simulink model "commande_position_axe"  (R2024b)
settings: Solver=VariableStepAuto  StartTime=0.0  StopTime=10.0  RelTol=1e-3
settings Model: Creator=firas  LastModifiedBy=firas

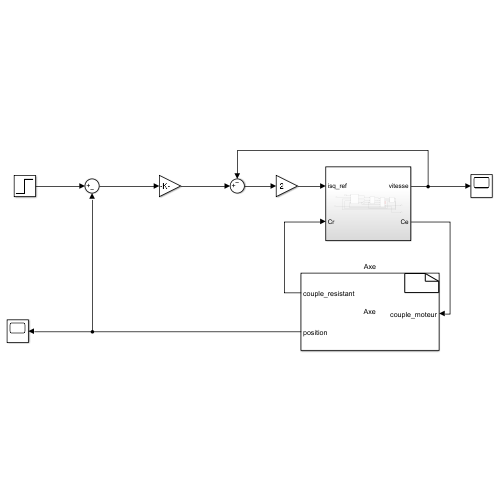
[thumbnail: Simulink's stored preview of the top-level diagram]
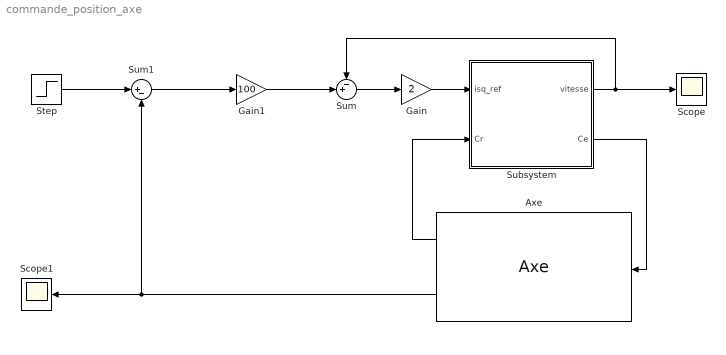
== system commande_position_axe ==
  Axe : S-Function  FunctionName=Axe  SFunctionModules=Axe_wrapper.c  SFunctionDeploymentMode=off  EnableBusSupport=off  mask(S-Function Builder){}
      mask help: Simulink:masks:SFunctionBuilder_MD
      mask init:
      | val = [[.9  0.75 0.75 1 1 .9 .9 1]',[1 1 0.75 0.75 .9 .9 1 .9]'];try , sys = get_param(gcb,'SfunBuilderFcnName');if isempty(sys), sys = get_param(gcb,'FunctionName'); end,catch, sys = get_param(gcb,'FunctionName'); end
      settings: CopyFcn=set_param(gcbh,'LinkStatus','none')  OpenFcn=sfunctionwizard(gcbh)
      mask Display:
      | plot(val(:,1),val(:,2))
      | disp(sys)
      | port_label('input',1,sprintf('%s', 'couple\_moteur'),'interpreter','tex')
      | port_label('output',1,sprintf('%s', 'couple\_resistant'),'interpreter','tex')
      | port_label('output',2,sprintf('%s', 'position'),'interpreter','tex')
  Gain : Gain  Gain=2
  Gain1 : Gain  Gain=100
  Scope : Scope
  Scope1 : Scope
  Step : Step  SampleTime=0
  Subsystem : Subsystem
  Sum : Sum  Inputs=-+|
  Sum1 : Sum  Inputs=|+-
  wires:
  Subsystem/2(Ce) -> Axe/1
  Axe/1 -> Subsystem/2(Cr)
  Sum/1 -> Gain/1
  Gain/1 -> Subsystem/1(isq_ref)
  Subsystem/1(vitesse) -> Scope/1, Sum/1
  Step/1 -> Sum1/1
  Axe/2 -> Sum1/2, Scope1/1
  Sum1/1 -> Gain1/1
  Gain1/1 -> Sum/2

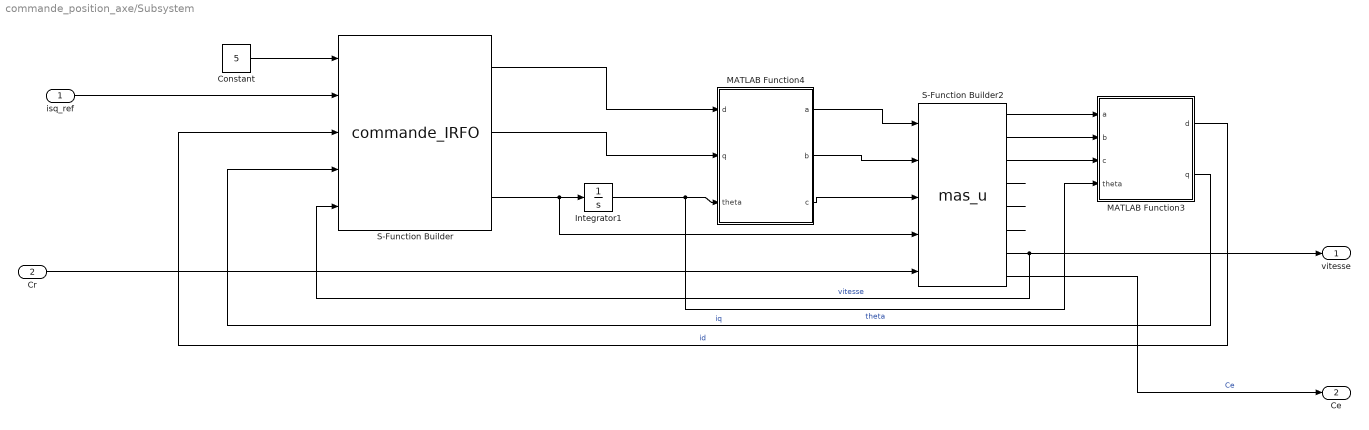
== system commande_position_axe/Subsystem ==
  isq_ref : Inport
  Cr : Inport  Port=2
  Constant : Constant  Value=5
  Integrator1 : Integrator
  MATLAB Function3 : MATLAB Function  TreatAsAtomicUnit=on
  MATLAB Function4 : MATLAB Function  TreatAsAtomicUnit=on
  S-Function Builder : S-Function  FunctionName=commande_IRFO  SFunctionModules=commande_IRFO_wrapper.c  SFunctionDeploymentMode=off  EnableBusSupport=off  mask(S-Function Builder){}
      mask help: Simulink:masks:SFunctionBuilder_MD
      mask init: same as commande_position_axe/Axe
      settings: CopyFcn=set_param(gcbh,'LinkStatus','none')  OpenFcn=sfunctionwizard(gcbh)
      mask Display:
      | plot(val(:,1),val(:,2))
      | disp(sys)
      | port_label('input',1,sprintf('%s', 'iphi\_ref'),'interpreter','tex')
      | port_label('input',2,sprintf('%s', 'isq\_ref'),'interpreter','tex')
      | port_label('input',3,sprintf('%s', 'isd'),'interpreter','tex')
      | port_label('input',4,sprintf('%s', 'isq'),'interpreter','tex')
      | port_label('input',5,sprintf('%s', 'vitesse'),'interpreter','tex')
      | port_label('output',1,sprintf('%s', 'vsd'),'interpreter','tex')
      | port_label('output',2,sprintf('%s', 'vsq'),'interpreter','tex')
      | port_label('output',3,sprintf('%s', 'ws'),'interpreter','tex')
  S-Function Builder2 : S-Function  FunctionName=mas_u  SFunctionModules=mas_u_wrapper.c  SFunctionDeploymentMode=off  EnableBusSupport=off  mask(S-Function Builder){}
      mask help: Simulink:masks:SFunctionBuilder_MD
      mask init: same as commande_position_axe/Axe
      settings: CopyFcn=set_param(gcbh,'LinkStatus','none')  OpenFcn=sfunctionwizard(gcbh)
      mask Display:
      | plot(val(:,1),val(:,2))
      | disp(sys)
      | port_label('input',1,sprintf('%s', 'vsa'),'interpreter','tex')
      | port_label('input',2,sprintf('%s', 'vsb'),'interpreter','tex')
      | port_label('input',3,sprintf('%s', 'vsc'),'interpreter','tex')
      | port_label('input',4,sprintf('%s', 'ws'),'interpreter','tex')
      | port_label('input',5,sprintf('%s', 'Cr'),'interpreter','tex')
      | port_label('output',1,sprintf('%s', 'isa'),'interpreter','tex')
      | port_label('output',2,sprintf('%s', 'isb'),'interpreter','tex')
      | port_label('output',3,sprintf('%s', 'isc'),'interpreter','tex')
      | port_label('output',4,sprintf('%s', 'ira'),'interpreter','tex')
      | port_label('output',5,sprintf('%s', 'irb'),'interpreter','tex')
      | port_label('output',6,sprintf('%s', 'irc'),'interpreter','tex')
      | port_label('output',7,sprintf('%s', 'vitesse'),'interpreter','tex')
      | port_label('output',8,sprintf('%s', 'Ce'),'interpreter','tex')
  vitesse : Outport
  Ce : Outport  Port=2
  wires:
  S-Function Builder2/4 -> ?
  S-Function Builder/2 -> MATLAB Function4/2(q)
  Integrator1/1 -> MATLAB Function4/3(theta), MATLAB Function3/4(theta)  "theta"
  S-Function Builder2/5 -> ?
  S-Function Builder/3 -> S-Function Builder2/4, Integrator1/1
  S-Function Builder2/1 -> MATLAB Function3/1(a)
  S-Function Builder2/7 -> vitesse/1, S-Function Builder/5  "vitesse"
  MATLAB Function3/1(d) -> S-Function Builder/3  "id"
  S-Function Builder2/2 -> MATLAB Function3/2(b)
  MATLAB Function4/1(a) -> S-Function Builder2/1
  S-Function Builder2/3 -> MATLAB Function3/3(c)
  Cr/1 -> S-Function Builder2/5
  MATLAB Function4/3(c) -> S-Function Builder2/3
  Constant/1 -> S-Function Builder/1
  S-Function Builder/1 -> MATLAB Function4/1(d)
  MATLAB Function3/2(q) -> S-Function Builder/4  "iq"
  MATLAB Function4/2(b) -> S-Function Builder2/2
  isq_ref/1 -> S-Function Builder/2
  S-Function Builder2/6 -> ?
  S-Function Builder2/8 -> Ce/1  "Ce"

== matlab function commande_position_axe/Subsystem/MATLAB Function3 ==
  data: a input; d output; b input; c input; theta input; q output
function [d,q] = Park_direct(a,b,c,theta)
    
     d = sqrt(2/3)*[cos(theta),cos(theta-2*pi/3),cos(theta+2*pi/3)]*[a;b;c];
     q = sqrt(2/3)*[-sin(theta),-sin(theta -2*pi/3),-sin(theta +2*pi/3)]*[a ; b ; c];
    
end

== matlab function commande_position_axe/Subsystem/MATLAB Function4 ==
  data: d input; a output; q input; theta input; b output; c output
function [a,b,c] = inverse_Park(d,q,theta)
    a = sqrt(2/3)*[cos(theta) -sin(theta)]*[d;q];
    b = sqrt(2/3)*[cos(theta-2*pi/3) -sin(theta-2*pi/3)]*[d;q];
    c = sqrt(2/3)*[cos(theta+2*pi/3) -sin(theta+2*pi/3)]*[d;q];
end
